simulink model "goertzel1"  (Simulink 7.0)
settings: Solver=ode45  StartTime=0.0  StopTime=50  RelTol=1e-3
libraries: dspbuff3 x1, dspwin32 x1
settings Model: Creator=fradet  LastModifiedBy=fradet

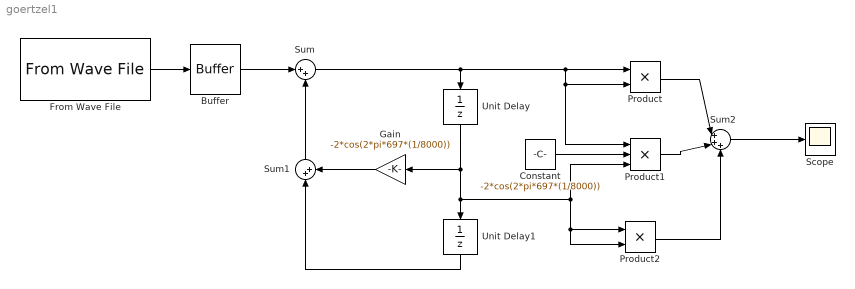
== system goertzel1 ==
  Buffer : dspbuff3/Buffer  N=1  V=0  ic=0
  Constant : Constant  Value=-2*cos(2*pi*697*(1/8000))  OutDataType=sfix(16)  OutScaling=2^0
  From Wave File : dspwin32/From Wave File  FileName=NumeroBE.wav  SamplesPerFrame=256  MinBufSize=256  dType=double  bLoop=off  timesToPlay=1  restartMode=immediately after last sample  firstSampleOutput=off  lastSampleOutput=off
  Gain : Gain  Orientation=left  Gain=-2*cos(2*pi*697*(1/8000))  ParameterDataType=sfix(16)  ParameterScaling=2^0  OutDataType=sfix(16)  OutScaling=2^0  SampleTime=1/8000
  Product : Product  OutDataType=sfix(16)  OutScaling=2^0  RndMeth=Zero
  Product1 : Product  Inputs=3  OutDataType=sfix(16)  OutScaling=2^0  RndMeth=Zero
  Product2 : Product  OutDataType=sfix(16)  OutScaling=2^0  RndMeth=Zero
  Scope : Scope
  Sum : Sum  Inputs=|++  OutDataType=sfix(16)  OutScaling=2^0
  Sum1 : Sum  Orientation=up  Inputs=|++  OutDataType=sfix(16)  OutScaling=2^0
  Sum2 : Sum  Inputs=|+++  OutDataType=sfix(16)  OutScaling=2^0
  Unit Delay : UnitDelay  Orientation=down
  Unit Delay1 : UnitDelay  Orientation=down
  wires:
  Unit Delay/1 -> Gain/1, Unit Delay1/1, Product1/3, Product2/1, Product2/2
  Sum/1 -> Unit Delay/1, Product/1, Product/2, Product1/1
  Unit Delay1/1 -> Sum1/1
  Gain/1 -> Sum1/2
  Sum1/1 -> Sum/2
  Constant/1 -> Product1/2
  Product/1 -> Sum2/1
  Product1/1 -> Sum2/2
  Product2/1 -> Sum2/3
  Sum2/1 -> Scope/1
  Buffer/1 -> Sum/1
  From Wave File/1 -> Buffer/1
